simulink model "model"  (R2015b)
settings: Solver=ode4  StartTime=0.0  StopTime=inf  FixedStep=0.01  RelTol=1e-3
undefined symbols (not defined in the file): Standard_Devices, UDP_Protocol
libraries: sldrtlib x2
settings Model: Creator=admin  LastModifiedBy=admin
settings HardwareCC: ProdBitPerLong=64  ProdLargestAtomicFloat=None  ProdHWDeviceType=Intel->x86-64  TargetBitPerLong=64  TargetBitPerPointer=64  TargetIntDivRoundTo=Zero  TargetEndianess=LittleEndian  TargetWordSize=64  TargetHWDeviceType=Intel->x86-64
settings RTWCC: SystemTargetFile=sldrt.tlc  TemplateMakefile=sldrt.tmf  Description=Simulink Desktop Real-Time  RTWCompilerOptimization=on
settings CodeAppCC: MaxIdLength=95
settings SimulinkDesktopRealTimeCC: TargetPreCompLibLocation=C:\Program Files\MATLAB\R2015b\toolbox\sldrt\lib\win64  TargetLangStandard=C89/C90 (ANSI)  SupportVariableSizeSignals=off

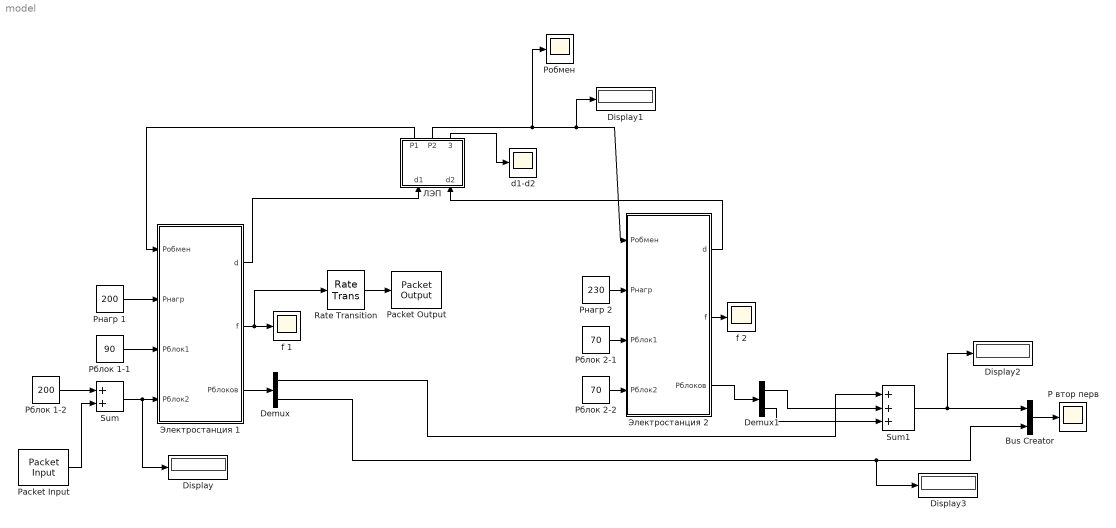
== system model ==
  Bus Creator : BusCreator  Inputs=2
  Demux : Demux  Outputs=2
  Demux1 : Demux  Outputs=2
  Display{,1..3} (4 alike) : Display
  P втор перв : Scope
  Packet Input : sldrtlib/Packet Input  SampleTime=0.01  MaxMissedTicks=1000  ShowMissedTicks=off  YieldWhenWaiting=off  DrvName=Standard_Devices/UDP_Protocol  DrvAddress=12000  DrvOptions=[182255628 12001]  PacketSize=8  DataTypes='1*double'  ShowReady=off  ShowError=off  PacketID=1  ByteOrder=1  ShowTimestamp=off
      settings: AttributesFormatString=Standard Devices\nUDP Protocol [2EE0h]
  Packet Output : sldrtlib/Packet Output  SampleTime=1  MaxMissedTicks=10  ShowMissedTicks=off  YieldWhenWaiting=off  DrvName=Standard_Devices/UDP_Protocol  DrvAddress=12000  DrvOptions=[182255628 12001]  PacketSize=8  DataTypes='1*double'  ShowReady=off  ShowError=off  PacketID=1  ByteOrder=1  InitialValue=[]  FinalValue=[]
      settings: AttributesFormatString=Standard Devices\nUDP Protocol [2EE0h]
  Pблок 1-1 : Constant  Value=90
  Pблок 1-2 : Constant  Value=200
  Pблок 2-1 : Constant  Value=70
  Pблок 2-2 : Constant  Value=70
  Pнагр 1 : Constant  Value=200
  Pнагр 2 : Constant  Value=230
  Pобмен : Scope
  Rate Transition : RateTransition  OutPortSampleTime=1
  Sum : Sum
  Sum1 : Sum  Inputs=+++
  d1-d2 : Scope
  f 1 : Scope
  f 2 : Scope
  ЛЭП : Subsystem
  Электростанция 1 : Subsystem
  Электростанция 2 : Subsystem
  wires:
  Rate Transition/1 -> Packet Output/1
  Электростанция 1/3(Pблоков) -> Demux/1
  Электростанция 1/2(f) -> Rate Transition/1, f 1/1
  Pнагр 1/1 -> Электростанция 1/2(Pнагр)
  Pблок 1-1/1 -> Электростанция 1/3(Pблок1)
  Pнагр 2/1 -> Электростанция 2/2(Pнагр)
  Pблок 2-2/1 -> Электростанция 2/4(Pблок2)
  Электростанция 2/2(f) -> f 2/1
  Электростанция 2/3(Pблоков) -> Demux1/1
  Электростанция 2/1(d) -> ЛЭП/2(d2)
  Электростанция 1/1(d) -> ЛЭП/1(d1)
  ЛЭП/2(P2) -> Pобмен/1, Display1/1, Электростанция 2/1(Pобмен)
  ЛЭП/1(P1) -> Электростанция 1/1(Pобмен)
  ЛЭП/3(d1-d2) -> d1-d2/1
  Pблок 2-1/1 -> Электростанция 2/3(Pблок1)
  Sum/1 -> Display/1, Электростанция 1/4(Pблок2)
  Pблок 1-2/1 -> Sum/1
  Packet Input/1 -> Sum/2
  Demux1/1 -> Sum1/2
  Demux1/2 -> Sum1/3
  Sum1/1 -> Display2/1, Bus Creator/1
  Demux/1 -> Sum1/1
  Demux/2 -> Display3/1, Bus Creator/2
  Bus Creator/1 -> P втор перв/1

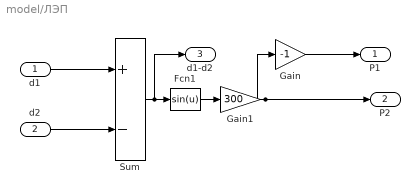
== system model/ЛЭП ==
  d1 : Inport
  d2 : Inport  Port=2
  Fcn1 : Fcn  Expr=sin(u)
  Gain : Gain  Gain=-1
  Gain1 : Gain  Gain=300
  Sum : Sum  Inputs=+-
  P1 : Outport
  P2 : Outport  Port=2
  d1-d2 : Outport  Port=3
  wires:
  Gain/1 -> P1/1
  Sum/1 -> d1-d2/1, Fcn1/1
  Gain1/1 -> Gain/1, P2/1
  d2/1 -> Sum/2
  Fcn1/1 -> Gain1/1
  d1/1 -> Sum/1

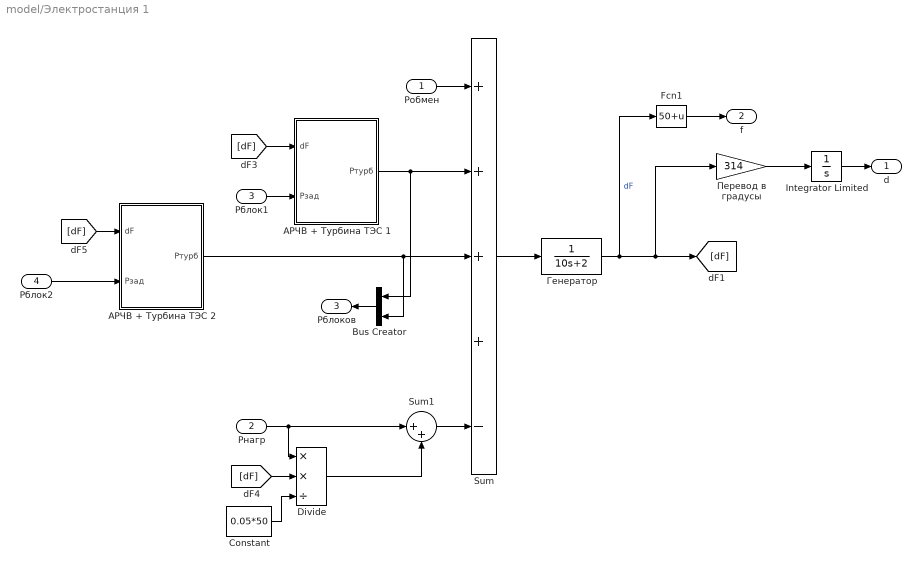
== system model/Электростанция 1 ==
  Pобмен : Inport
  Pнагр : Inport  Port=2
  Pблок1 : Inport  Port=3
  Pблок2 : Inport  Port=4
  Bus Creator : BusCreator  Inputs=2
  Constant : Constant  Value=0.05*50
  Divide : Product  Inputs=**/
  Fcn1 : Fcn  Expr=50+u
  Integrator Limited : Integrator  UpperSaturationLimit=180  LowerSaturationLimit=-180  WrapState=on
  Sum : Sum  Inputs=++++-
  Sum1 : Sum  Inputs=|++
  АРЧВ + Турбина ТЭС 1 : Subsystem  mask{Pnom=200, Droop=0.05}
      mask prompts: Pnom "Pном"; Droop "Статизм"
  АРЧВ + Турбина ТЭС 2 : Subsystem  mask{Pnom=400, Droop=0.05}
      mask prompts: Pnom "Pном"; Droop "Статизм"
  Генератор : TransferFcn  Denominator=[10 2]
  Перевод в градусы : Gain  Gain=314
  d : Outport
  f : Outport  Port=2
  Pблоков : Outport  Port=3
  wires:
  Sum/1 -> Генератор/1
  Pблок2/1 -> АРЧВ + Турбина ТЭС 2/2(Pзад)
  АРЧВ + Турбина ТЭС 2/1(Pтурб) -> Sum/3, Bus Creator/2
  Sum1/1 -> Sum/5
  Pобмен/1 -> Sum/1
  Pблок1/1 -> АРЧВ + Турбина ТЭС 1/2(Pзад)
  Генератор/1 -> Fcn1/1, Перевод в градусы/1, [dF]  "dF"
  [dF] -> АРЧВ + Турбина ТЭС 2/1(dF)
  [dF] -> АРЧВ + Турбина ТЭС 1/1(dF)
  Pнагр/1 -> Divide/1, Sum1/1
  Fcn1/1 -> f/1
  Bus Creator/1 -> Pблоков/1
  Перевод в градусы/1 -> Integrator Limited/1
  Integrator Limited/1 -> d/1
  Constant/1 -> Divide/3
  [dF] -> Divide/2
  Divide/1 -> Sum1/2
  АРЧВ + Турбина ТЭС 1/1(Pтурб) -> Bus Creator/1, Sum/2

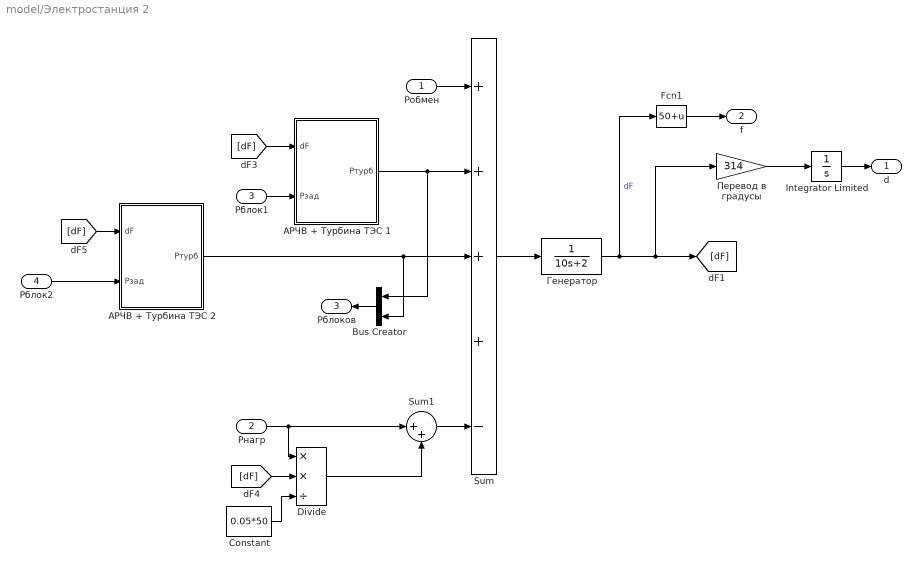
== system model/Электростанция 2 ==
  Pобмен : Inport
  Pнагр : Inport  Port=2
  Pблок1 : Inport  Port=3
  Pблок2 : Inport  Port=4
  Bus Creator : BusCreator  Inputs=2
  Constant : Constant  Value=0.05*50
  Divide : Product  Inputs=**/
  Fcn1 : Fcn  Expr=50+u
  Integrator Limited : Integrator  UpperSaturationLimit=180  LowerSaturationLimit=-180  WrapState=on
  Sum : Sum  Inputs=++++-
  Sum1 : Sum  Inputs=|++
  АРЧВ + Турбина ТЭС 1 : Subsystem  mask{Pnom=200, Droop=0.05}
      mask prompts: Pnom "Pном"; Droop "Статизм"
  АРЧВ + Турбина ТЭС 2 : Subsystem  mask{Pnom=200, Droop=0.05}
      mask prompts: Pnom "Pном"; Droop "Статизм"
  Генератор : TransferFcn  Denominator=[10 2]
  Перевод в градусы : Gain  Gain=314
  d : Outport
  f : Outport  Port=2
  Pблоков : Outport  Port=3
  wires:
  Sum/1 -> Генератор/1
  Pблок2/1 -> АРЧВ + Турбина ТЭС 2/2(Pзад)
  АРЧВ + Турбина ТЭС 2/1(Pтурб) -> Sum/3, Bus Creator/2
  Sum1/1 -> Sum/5
  Pобмен/1 -> Sum/1
  Pблок1/1 -> АРЧВ + Турбина ТЭС 1/2(Pзад)
  Генератор/1 -> Fcn1/1, Перевод в градусы/1, [dF]  "dF"
  [dF] -> АРЧВ + Турбина ТЭС 2/1(dF)
  [dF] -> АРЧВ + Турбина ТЭС 1/1(dF)
  Pнагр/1 -> Divide/1, Sum1/1
  Fcn1/1 -> f/1
  Bus Creator/1 -> Pблоков/1
  Перевод в градусы/1 -> Integrator Limited/1
  Integrator Limited/1 -> d/1
  Constant/1 -> Divide/3
  [dF] -> Divide/2
  Divide/1 -> Sum1/2
  АРЧВ + Турбина ТЭС 1/1(Pтурб) -> Bus Creator/1, Sum/2

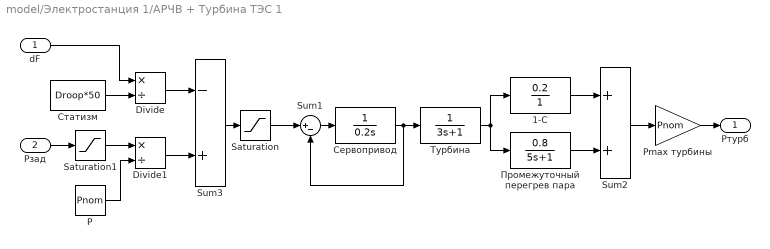
== system model/Электростанция 1/АРЧВ + Турбина ТЭС 1 ==
  dF : Inport
  Pзад : Inport  Port=2
  1-С : TransferFcn  Numerator=[0.2]  Denominator=[0 1]
  Divide : Product  Inputs=*/
  Divide1 : Product  Inputs=*/
  P : Constant  Value=Pnom
  Pmax турбины : Gain  Gain=Pnom
  Saturation : Saturate  UpperLimit=1  LowerLimit=0
  Saturation1 : Saturate  UpperLimit=Pnom  LowerLimit=0
  Sum1 : Sum  Inputs=|+-
  Sum2 : Sum
  Sum3 : Sum  Inputs=-+
  Промежуточный перегрев пара : TransferFcn  Numerator=[0.8]  Denominator=[5 1]
  Сервопривод : TransferFcn  Denominator=[0.2 0]
  Статизм : Constant  Value=Droop*50
  Турбина : TransferFcn  Denominator=[3 1]
  Pтурб : Outport
  wires:
  Pзад/1 -> Saturation1/1
  Saturation1/1 -> Divide1/1
  Divide1/1 -> Sum3/2
  dF/1 -> Divide/1
  P/1 -> Divide1/2
  Sum3/1 -> Saturation/1
  Промежуточный перегрев пара/1 -> Sum2/2
  Статизм/1 -> Divide/2
  Sum1/1 -> Сервопривод/1
  Турбина/1 -> 1-С/1, Промежуточный перегрев пара/1
  Сервопривод/1 -> Турбина/1, Sum1/2
  1-С/1 -> Sum2/1
  Sum2/1 -> Pmax турбины/1
  Divide/1 -> Sum3/1
  Saturation/1 -> Sum1/1
  Pmax турбины/1 -> Pтурб/1

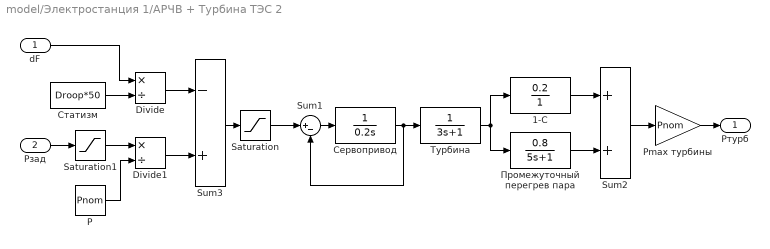
== system model/Электростанция 1/АРЧВ + Турбина ТЭС 2 ==
  dF : Inport
  Pзад : Inport  Port=2
  1-С : TransferFcn  Numerator=[0.2]  Denominator=[0 1]
  Divide : Product  Inputs=*/
  Divide1 : Product  Inputs=*/
  P : Constant  Value=Pnom
  Pmax турбины : Gain  Gain=Pnom
  Saturation : Saturate  UpperLimit=1  LowerLimit=0
  Saturation1 : Saturate  UpperLimit=Pnom  LowerLimit=0
  Sum1 : Sum  Inputs=|+-
  Sum2 : Sum
  Sum3 : Sum  Inputs=-+
  Промежуточный перегрев пара : TransferFcn  Numerator=[0.8]  Denominator=[5 1]
  Сервопривод : TransferFcn  Denominator=[0.2 0]
  Статизм : Constant  Value=Droop*50
  Турбина : TransferFcn  Denominator=[3 1]
  Pтурб : Outport
  wires:
  Pзад/1 -> Saturation1/1
  Saturation1/1 -> Divide1/1
  Divide1/1 -> Sum3/2
  dF/1 -> Divide/1
  P/1 -> Divide1/2
  Sum3/1 -> Saturation/1
  Промежуточный перегрев пара/1 -> Sum2/2
  Статизм/1 -> Divide/2
  Sum1/1 -> Сервопривод/1
  Турбина/1 -> 1-С/1, Промежуточный перегрев пара/1
  Сервопривод/1 -> Турбина/1, Sum1/2
  1-С/1 -> Sum2/1
  Sum2/1 -> Pmax турбины/1
  Divide/1 -> Sum3/1
  Saturation/1 -> Sum1/1
  Pmax турбины/1 -> Pтурб/1

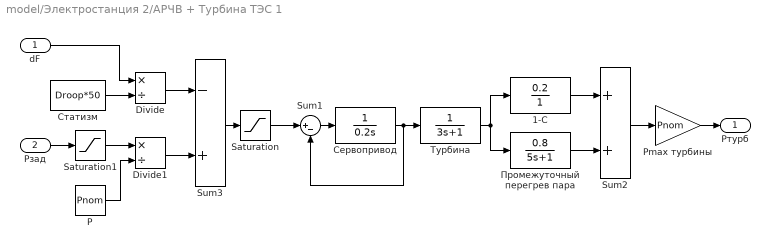
== system model/Электростанция 2/АРЧВ + Турбина ТЭС 1 ==
  dF : Inport
  Pзад : Inport  Port=2
  1-С : TransferFcn  Numerator=[0.2]  Denominator=[0 1]
  Divide : Product  Inputs=*/
  Divide1 : Product  Inputs=*/
  P : Constant  Value=Pnom
  Pmax турбины : Gain  Gain=Pnom
  Saturation : Saturate  UpperLimit=1  LowerLimit=0
  Saturation1 : Saturate  UpperLimit=Pnom  LowerLimit=0
  Sum1 : Sum  Inputs=|+-
  Sum2 : Sum
  Sum3 : Sum  Inputs=-+
  Промежуточный перегрев пара : TransferFcn  Numerator=[0.8]  Denominator=[5 1]
  Сервопривод : TransferFcn  Denominator=[0.2 0]
  Статизм : Constant  Value=Droop*50
  Турбина : TransferFcn  Denominator=[3 1]
  Pтурб : Outport
  wires:
  Pзад/1 -> Saturation1/1
  Saturation1/1 -> Divide1/1
  Divide1/1 -> Sum3/2
  dF/1 -> Divide/1
  P/1 -> Divide1/2
  Sum3/1 -> Saturation/1
  Промежуточный перегрев пара/1 -> Sum2/2
  Статизм/1 -> Divide/2
  Sum1/1 -> Сервопривод/1
  Турбина/1 -> 1-С/1, Промежуточный перегрев пара/1
  Сервопривод/1 -> Турбина/1, Sum1/2
  1-С/1 -> Sum2/1
  Sum2/1 -> Pmax турбины/1
  Divide/1 -> Sum3/1
  Saturation/1 -> Sum1/1
  Pmax турбины/1 -> Pтурб/1

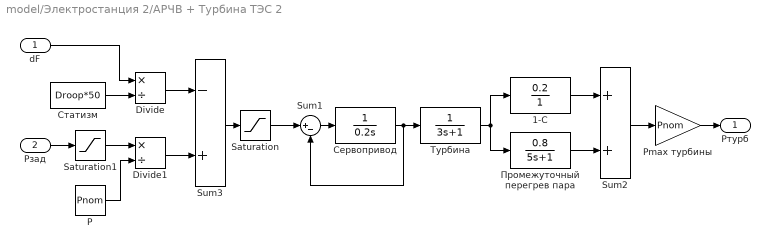
== system model/Электростанция 2/АРЧВ + Турбина ТЭС 2 ==
  dF : Inport
  Pзад : Inport  Port=2
  1-С : TransferFcn  Numerator=[0.2]  Denominator=[0 1]
  Divide : Product  Inputs=*/
  Divide1 : Product  Inputs=*/
  P : Constant  Value=Pnom
  Pmax турбины : Gain  Gain=Pnom
  Saturation : Saturate  UpperLimit=1  LowerLimit=0
  Saturation1 : Saturate  UpperLimit=Pnom  LowerLimit=0
  Sum1 : Sum  Inputs=|+-
  Sum2 : Sum
  Sum3 : Sum  Inputs=-+
  Промежуточный перегрев пара : TransferFcn  Numerator=[0.8]  Denominator=[5 1]
  Сервопривод : TransferFcn  Denominator=[0.2 0]
  Статизм : Constant  Value=Droop*50
  Турбина : TransferFcn  Denominator=[3 1]
  Pтурб : Outport
  wires:
  Pзад/1 -> Saturation1/1
  Saturation1/1 -> Divide1/1
  Divide1/1 -> Sum3/2
  dF/1 -> Divide/1
  P/1 -> Divide1/2
  Sum3/1 -> Saturation/1
  Промежуточный перегрев пара/1 -> Sum2/2
  Статизм/1 -> Divide/2
  Sum1/1 -> Сервопривод/1
  Турбина/1 -> 1-С/1, Промежуточный перегрев пара/1
  Сервопривод/1 -> Турбина/1, Sum1/2
  1-С/1 -> Sum2/1
  Sum2/1 -> Pmax турбины/1
  Divide/1 -> Sum3/1
  Saturation/1 -> Sum1/1
  Pmax турбины/1 -> Pтурб/1
